simulink model "pTMS"  (R2023b)
settings: Solver=VariableStepAuto  StartTime=0.0  StopTime=.05  RelTol=1e-3
undefined symbols (not defined in the file or in its folder): sawtooth
libraries: fl_lib x11, nesl_utility x10, simulink x3, ee_lib x1
settings Model: Creator=toren  LastModifiedBy=torenarginteanu

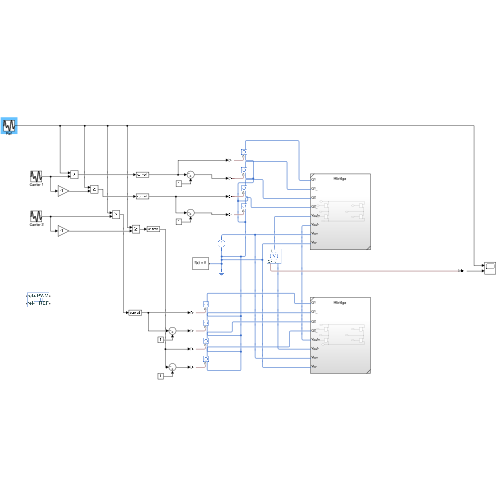
[thumbnail: Simulink's stored preview of the top-level diagram]
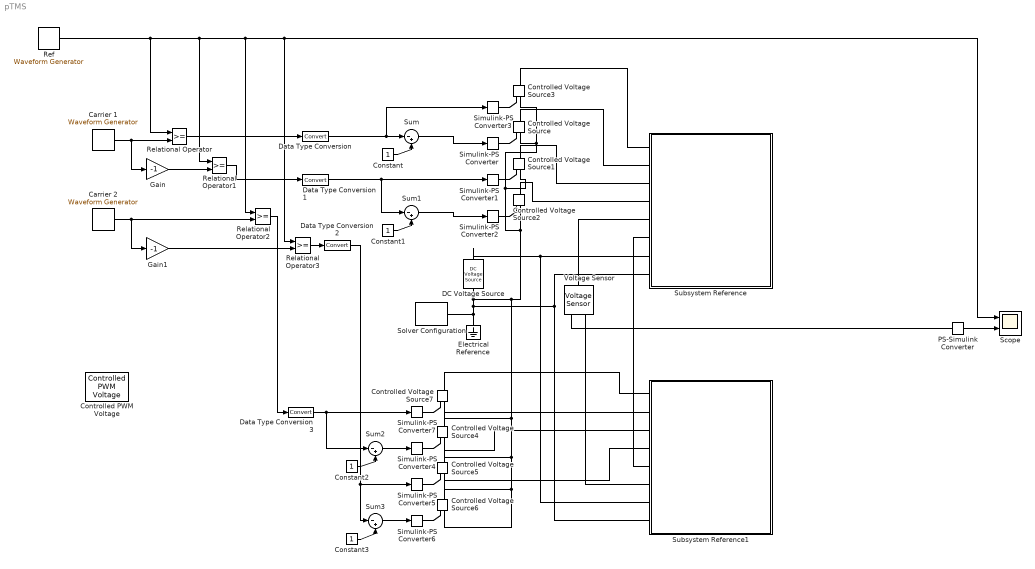
== system pTMS ==
  " Carrier 1" : simulink/Sources/Waveform Generator  OutMin=[]  OutMax=[]  OutDataTypeStr=double  SelectedSignal=1  Signals=sawtooth('Amplitude',1,'Frequency',2*pi*10000,'Phase',0)  BlockNames=MultiportSwitch_360967eb130d4fd  SampleTime=1e-6
  " Carrier 2" : simulink/Sources/Waveform Generator  OutMin=[]  OutMax=[]  OutDataTypeStr=double  SelectedSignal=1  Signals=sawtooth('Amplitude',1,'Frequency',2*pi*10000,'Phase',pi/2)  BlockNames=MultiportSwitch_75336a6b5fed493  SampleTime=1e-6
  Constant{,1..3} (4 alike) : Constant
  Controlled PWM Voltage : ee_lib/Integrated Circuits/Controlled PWM Voltage  F=1000 Hz  TD=0 s  pulse_width_offset=0 s  pulse_min=0 s  pwm_or_av=ee.enum.pwm_or_av.pwm  event_type=ee.enum.ic.event.asynchronous  sample_time=1e-6 s  Vmin=0 V  Vmax=5 V  Vm=5 V  u_min=0  u_max=1
  Controlled Voltage Source{,1..7} (8 alike) : fl_lib/Electrical/Electrical Sources/Controlled Voltage Source
  DC Voltage Source : fl_lib/Electrical/Electrical Sources/DC Voltage Source  v0=120 V
  Data Type Conversion{,1..3} (4 alike) : DataTypeConversion  SaturateOnIntegerOverflow=off  RndMeth=Floor
  Electrical Reference : fl_lib/Electrical/Electrical Elements/Electrical Reference
  Gain : Gain  Gain=-1
  Gain1 : Gain  Gain=-1
  PS-Simulink Converter : nesl_utility/PS-Simulink Converter  PhysicalDomain=network_engine_domain  SubClassName=ps_output  LeftPortType=input  RightPortType=output  PseudoPeriodic=off  Frequencies=[]  VectorFormat=inherit  Unit=inherit  AffineConversion=off
  Ref : simulink/Sources/Waveform Generator  OutMin=[]  OutMax=[]  OutDataTypeStr=double  SelectedSignal=1  Signals=sin('Amplitude',1,'Frequency',2*pi*100,'Phase',0)  BlockNames=MultiportSwitch_9436d083ac3d4e2  SampleTime=1e-6
  Relational Operator : RelationalOperator  OutDataTypeStr=fixdt(1,16)  RndMeth=Simplest  InputSameDT=off
  Relational Operator1 : RelationalOperator  OutDataTypeStr=boolean  RndMeth=Simplest  InputSameDT=off
  Relational Operator2 : RelationalOperator  OutDataTypeStr=boolean  RndMeth=Simplest  InputSameDT=off
  Relational Operator3 : RelationalOperator  OutDataTypeStr=boolean  RndMeth=Simplest  InputSameDT=off
  Scope : Scope  NumInputPorts=2
  Simulink-PS Converter{,1..7} (8 alike) : nesl_utility/Simulink-PS Converter  PhysicalDomain=network_engine_domain  SubClassName=ps_input  LeftPortType=input  RightPortType=output  PseudoPeriodic=off  Frequencies=[]  NoiseDistribution=none  NoiseParameters=[]  Unit=1  AffineConversion=off  FilteringAndDerivatives=provide  SimscapeFilterOrder=1  InputFilterTimeConstant=0.001  UdotUserProvided=0
  Solver Configuration : nesl_utility/Solver Configuration  PhysicalDomain=network_engine_domain  SubClassName=solver  LeftPortType=input  RightPortType=generic  Tones=[]  Harmonics=[]  SimulateNoise=off  Profile=off  UseLocalSampling=off  EnableSwitchedLinearOptims=on  FrequencyDomain=off  UseCCode=off  RelTol=0.001  AbsTol=0.001  MinStep=1e-09  ToWorkspace=off  RevertToSquareIcSolve=off  NumHomotopyIterations=100  PhasorMode=off  PhasorModeNumHarmonics=1  ConsistencySolver=NEWTON_XTOL_AFTER_FTOL  IndexReductionMethod=DerivativeReplacement  DoDC=off  ResidualTolerance=1e-09  ConsistencyTolSource=GLOBAL  ConsistencyAbsTol=0.001  ConsistencyRelTol=0.001  ConsistencyTolFactor=0.001  UseLocalSolver=off  LocalSolverChoice=NE_BACKWARD_EULER_ADVANCER  ResolveIndetEquations=on  FunctionEvalNumThread=1  LocalSolverSampleTime=0.001  DoFixedCost=off  MaxNonlinIter=3  MaxModeIter=2  ComputeImpulses=off  ImpulseIterations=2  LinearAlgebra=auto  LinearAlgebraNumThread=0  EquationFormulation=NE_TIME_EF  DelaysMemoryBudget=1024  AutomaticFiltering=on  FilteringTimeConstant=0.001  PartitionStorageMethod=AS_NEEDED  PartitionMemoryBudget=1024  PartitionMethod=ROBUST  MultibodyUseLocalSolver=off  MultibodyLocalSolverChoice=ODE1  MultibodyLocalSolverSampleTime=0.001
  Subsystem Reference : Subsystem  ReferencedSubsystem=Hbridge
  Subsystem Reference1 : Subsystem  ReferencedSubsystem=Hbridge
  Sum{,1..3} (4 alike) : Sum  Inputs=|-+
  Voltage Sensor : fl_lib/Electrical/Electrical Sensors/Voltage Sensor
  wires:
  PS-Simulink Converter/1 -> Scope/2
  Ref/1 -> Relational Operator/1, Relational Operator1/1, Relational Operator2/1, Relational Operator3/1, Scope/1
  " Carrier 1"/1 -> Relational Operator/2, Gain/1
  " Carrier 2"/1 -> Relational Operator2/2, Gain1/1
  Gain/1 -> Relational Operator1/2
  Gain1/1 -> Relational Operator3/2
  Relational Operator/1 -> Data Type Conversion/1
  Constant/1 -> Sum/2
  Sum/1 -> Simulink-PS Converter/1
  Relational Operator1/1 -> Data Type Conversion1/1
  Constant1/1 -> Sum1/2
  Sum1/1 -> Simulink-PS Converter2/1
  Relational Operator3/1 -> Data Type Conversion2/1
  Relational Operator2/1 -> Data Type Conversion3/1
  Constant2/1 -> Sum2/2
  Constant3/1 -> Sum3/2
  Sum3/1 -> Simulink-PS Converter6/1
  Sum2/1 -> Simulink-PS Converter4/1
  Data Type Conversion/1 -> Sum/1, Simulink-PS Converter3/1
  Data Type Conversion1/1 -> Sum1/1, Simulink-PS Converter1/1
  Data Type Conversion2/1 -> Sum3/1, Simulink-PS Converter5/1
  Data Type Conversion3/1 -> Sum2/1, Simulink-PS Converter7/1
  connections:
  DC Voltage Source/LConn1 -- Subsystem Reference1/LConn7 -- Subsystem Reference/LConn7
  DC Voltage Source/RConn1 -- Controlled Voltage Source6/RConn2 -- Controlled Voltage Source5/RConn2 -- Controlled Voltage Source4/RConn2 -- Controlled Voltage Source7/RConn2 -- Controlled Voltage Source3/RConn2 -- Controlled Voltage Source/RConn2 -- Controlled Voltage Source1/RConn2 -- Controlled Voltage Source2/RConn2 -- Solver Configuration/RConn1 -- Electrical Reference/LConn1 -- Subsystem Reference/LConn8 -- Subsystem Reference1/LConn8
  Subsystem Reference1/LConn5 -- Subsystem Reference/LConn6
  Voltage Sensor/LConn1 -- Subsystem Reference/LConn5
  Voltage Sensor/RConn2 -- Subsystem Reference1/LConn6
  Voltage Sensor/RConn1 -- PS-Simulink Converter/LConn1
  Simulink-PS Converter/RConn1 -- Controlled Voltage Source/RConn1
  Simulink-PS Converter1/RConn1 -- Controlled Voltage Source1/RConn1
  Simulink-PS Converter2/RConn1 -- Controlled Voltage Source2/RConn1
  Simulink-PS Converter3/RConn1 -- Controlled Voltage Source3/RConn1
  Simulink-PS Converter4/RConn1 -- Controlled Voltage Source4/RConn1
  Simulink-PS Converter6/RConn1 -- Controlled Voltage Source6/RConn1
  Simulink-PS Converter5/RConn1 -- Controlled Voltage Source5/RConn1
  Simulink-PS Converter7/RConn1 -- Controlled Voltage Source7/RConn1
  Controlled Voltage Source2/LConn1 -- Subsystem Reference/LConn4
  Controlled Voltage Source1/LConn1 -- Subsystem Reference/LConn3
  Controlled Voltage Source/LConn1 -- Subsystem Reference/LConn2
  Controlled Voltage Source3/LConn1 -- Subsystem Reference/LConn1
  Controlled Voltage Source7/LConn1 -- Subsystem Reference1/LConn1
  Subsystem Reference1/LConn2 -- Controlled Voltage Source4/LConn1
  Controlled Voltage Source5/LConn1 -- Subsystem Reference1/LConn3
  Subsystem Reference1/LConn4 -- Controlled Voltage Source6/LConn1
